simulink model "userdefined_funtion_test_org"  (Simulink 10.0)
settings: Solver=ode45  StartTime=0.0  StopTime=10.0  RelTol=1e-3  EnableMultiTasking=on
settings Model: Creator=brownaa  LastModifiedBy=annonymous
settings DataIOCC: LimitDataPoints=on
settings DebuggingCC: UnderspecifiedInitializationDetection=Simplified  MergeDetectMultiDrivingBlocksExec=error  SolverPrmCheckMsg=warning
settings GRTTargetCC: GeneratePreprocessorConditionals=Disable all  CombineOutputUpdateFcns=on  GRTInterface=off
settings ConfigComp: CovExternalEMLEnable=off  CovSFcnEnable=off

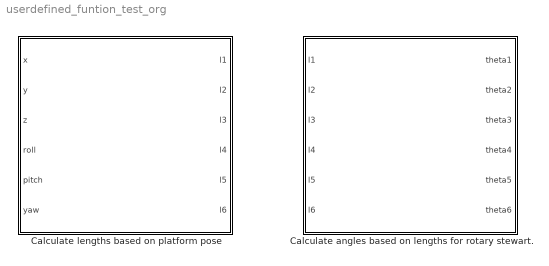
== system userdefined_funtion_test_org ==
  " Calculate angles based on lengths for rotary stewart." : MATLAB Function  TreatAsAtomicUnit=on
  Calculate lengths based on platform pose : MATLAB Function  TreatAsAtomicUnit=on

== matlab function Calculate lengths based on platform pose ==
  data: x input double; y input double; z input double; roll input double; pitch input double; yaw input double; l1 output double; l2 output double; l3 output double; l4 output double; l5 output double; l6 output double
function [l1,l2,l3,l4,l5,l6] = fcn(x,y,z,roll,pitch,yaw)
%#codegen

l1=0;
l2=0;
l3=0;
l4=0;
l5=0;
l6=0;
end

== matlab function  Calculate angles based on lengths for rotary stewart. ==
  data: l1 input double; l2 input double; l3 input double; l4 input double; l5 input double; l6 input double; theta1 output double; theta2 output double; theta3 output double; theta4 output double; theta5 output double; theta6 output double
function [theta1,theta2,theta3,theta4,theta5,theta6] = fcn(l1,l2,l3,l4,l5,l6)
%#codegen

l1=0;
l2=0;
l3=0;
l4=0;
l5=0;
l6=0;
end
